simulink model "incrementerdigital12"  (R2024a)
settings: Solver=VariableStepAuto  StartTime=0.0  StopTime=10.0  RelTol=1e-3
settings Model: Creator=tusha  LastModifiedBy=tusha

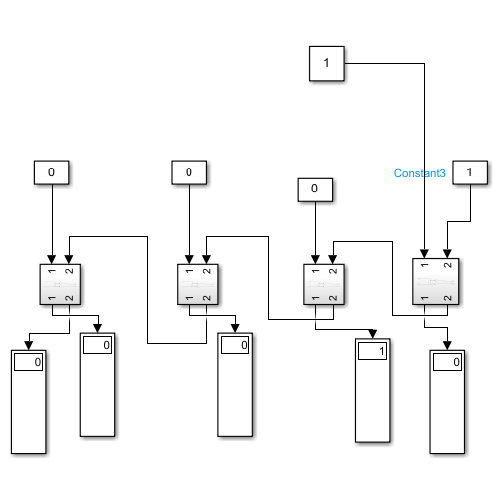
[thumbnail: Simulink's stored preview of the top-level diagram]
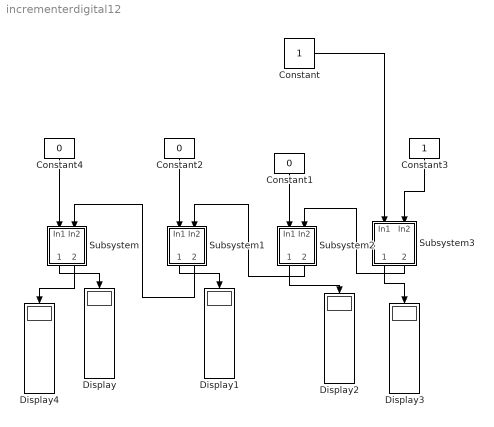
== system incrementerdigital12 ==
  Constant : Constant
  Constant1 : Constant  Value=0
  Constant2 : Constant  Value=0
  Constant3 : Constant
  Constant4 : Constant  Value=0
  Display{,1..4} (5 alike) : Display
  Subsystem : Subsystem
  Subsystem1 : Subsystem
  Subsystem2 : Subsystem
  Subsystem3 : Subsystem
  wires:
  Constant4/1 -> Subsystem/1(In1)
  Constant2/1 -> Subsystem1/1(In1)
  Constant1/1 -> Subsystem2/1(In1)
  Subsystem3/1(Out1) -> Display3/1
  Subsystem3/2(Out2) -> Subsystem2/2(In2)
  Constant3/1 -> Subsystem3/2(In2)
  Constant/1 -> Subsystem3/1(In1)
  Subsystem2/2(Out2) -> Subsystem1/2(In2)
  Subsystem2/1(Out1) -> Display2/1
  Subsystem1/1(Out1) -> Display1/1
  Subsystem1/2(Out2) -> Subsystem/2(In2)
  Subsystem/1(Out1) -> Display/1
  Subsystem/2(Out2) -> Display4/1

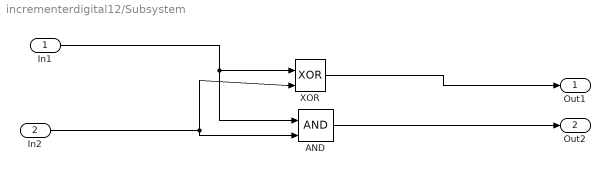
== system incrementerdigital12/Subsystem ==
  In1 : Inport
  In2 : Inport  Port=2
  AND : Logic  IconShape=distinctive  AllPortsSameDT=off  OutDataTypeStr=boolean
  XOR : Logic  Operator=XOR  IconShape=distinctive  AllPortsSameDT=off  OutDataTypeStr=boolean
  Out1 : Outport
  Out2 : Outport  Port=2
  wires:
  In1/1 -> AND/1, XOR/1
  In2/1 -> XOR/2, AND/2
  AND/1 -> Out2/1
  XOR/1 -> Out1/1

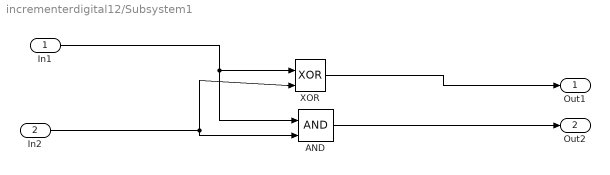
== system incrementerdigital12/Subsystem1 ==
  In1 : Inport
  In2 : Inport  Port=2
  AND : Logic  IconShape=distinctive  AllPortsSameDT=off  OutDataTypeStr=boolean
  XOR : Logic  Operator=XOR  IconShape=distinctive  AllPortsSameDT=off  OutDataTypeStr=boolean
  Out1 : Outport
  Out2 : Outport  Port=2
  wires:
  In1/1 -> AND/1, XOR/1
  In2/1 -> XOR/2, AND/2
  AND/1 -> Out2/1
  XOR/1 -> Out1/1

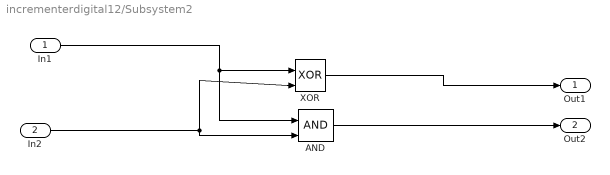
== system incrementerdigital12/Subsystem2 ==
  In1 : Inport
  In2 : Inport  Port=2
  AND : Logic  IconShape=distinctive  AllPortsSameDT=off  OutDataTypeStr=boolean
  XOR : Logic  Operator=XOR  IconShape=distinctive  AllPortsSameDT=off  OutDataTypeStr=boolean
  Out1 : Outport
  Out2 : Outport  Port=2
  wires:
  In1/1 -> AND/1, XOR/1
  In2/1 -> XOR/2, AND/2
  AND/1 -> Out2/1
  XOR/1 -> Out1/1

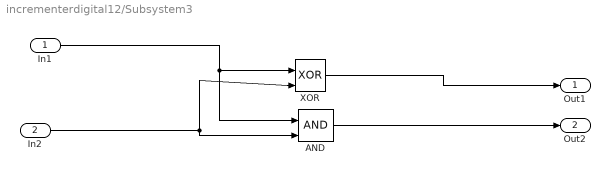
== system incrementerdigital12/Subsystem3 ==
  In1 : Inport
  In2 : Inport  Port=2
  AND : Logic  IconShape=distinctive  AllPortsSameDT=off  OutDataTypeStr=boolean
  XOR : Logic  Operator=XOR  IconShape=distinctive  AllPortsSameDT=off  OutDataTypeStr=boolean
  Out1 : Outport
  Out2 : Outport  Port=2
  wires:
  In1/1 -> AND/1, XOR/1
  In2/1 -> XOR/2, AND/2
  AND/1 -> Out2/1
  XOR/1 -> Out1/1
